simulink model "ss_model_dpt"  (R2021b)
settings: Solver=VariableStepAuto  StartTime=0.0  StopTime=0.3  RelTol=1e-3
undefined symbols (not defined in the file): Jn, ke, km, L, Mn, R
settings Model: Creator=vkad  LastModifiedBy=vkad

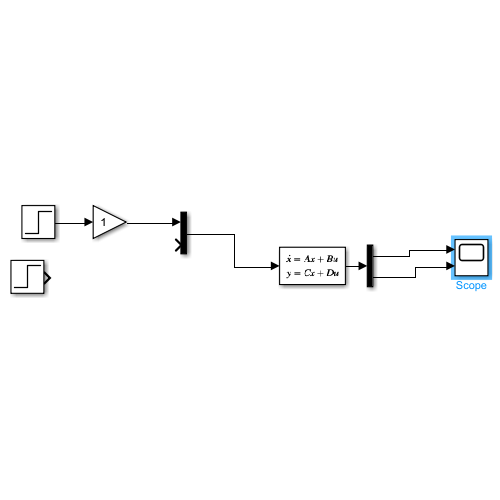
[thumbnail: Simulink's stored preview of the top-level diagram]
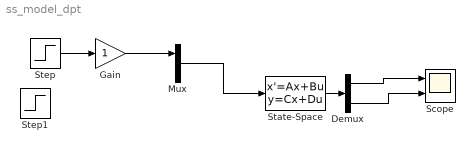
== system ss_model_dpt ==
  Demux : Demux  Outputs=2
  Gain : Gain
  Mux : Mux  Inputs=2
  Scope : Scope  NumInputPorts=2
  State-Space : StateSpace  A=[-R/L -ke/L; km/Jn 0]  B=[1/L 0; 0 -1/Jn]  C=[km 0; 0 1]  D=[0 0; 0 0]  InitialCondition=0
  Step : Step  Time=0  SampleTime=0
  Step1 : Step  Time=0  After=Mn  SampleTime=0
  wires:
  Mux/1 -> State-Space/1
  Gain/1 -> Mux/1
  Step/1 -> Gain/1
  State-Space/1 -> Demux/1
  Demux/1 -> Scope/1
  Demux/2 -> Scope/2
